simulink model "dspproject"  (R2025b)
settings: Solver=VariableStepAuto  StartTime=0.0  StopTime=10.0  RelTol=1e-3
undefined symbols (not defined in the file): dspblkCoreblockFVToolHelper, gcbh
libraries: audiofeatures x2, simulink x1, dspxfrm3 x1, dspsigops x1, dspvision x1
settings Model: Creator=BILMOOT  LastModifiedBy=BILMOOT

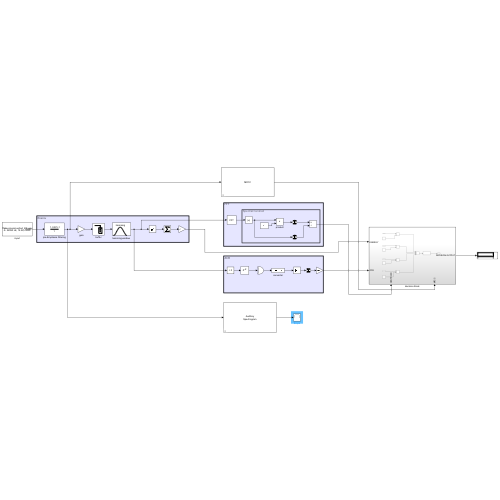
[thumbnail: Simulink's stored preview of the top-level diagram]
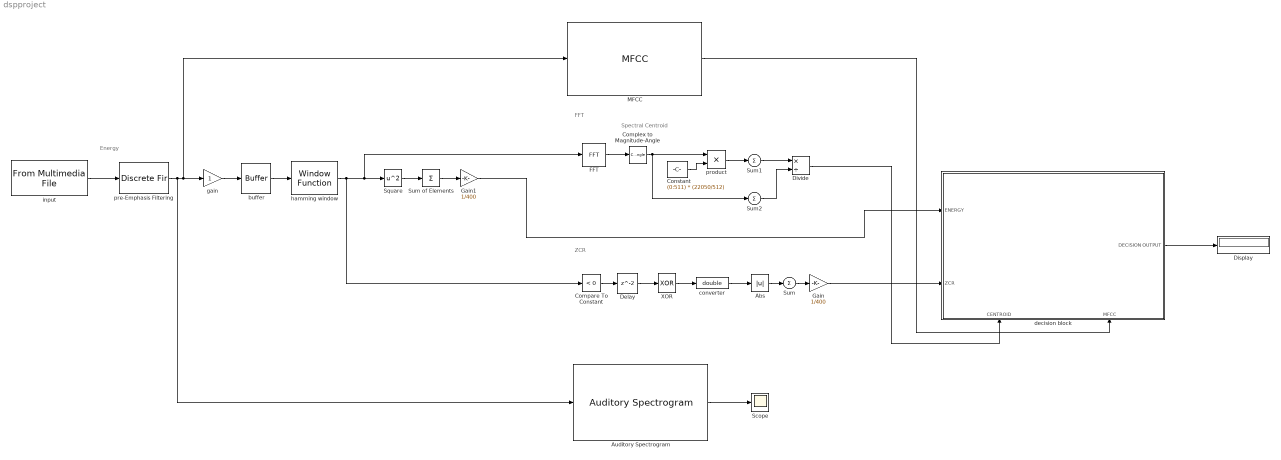
== system dspproject ==
  note: FFT
  note: Spectral Centroid
  note: Energy
  note: ZCR
  Abs : Abs  SaturateOnIntegerOverflow=off
  Auditory Spectrogram : audiofeatures/Auditory Spectrogram  FrequencyScale=mel  MelStyle=slaney  AutoNumBands=on  NumBands=32  AutoFrequencyRange=on  FrequencyRange=[0, 22050]  FilterBankDesignDomain=linear  FilterBankNormalization=bandwidth  OutputFrequencyVector=off  WindowParameter=hamming(400,'periodic')  WindowNormalization=on  OverlapLength=200  AutoFFTLength=on  FFTLength=1024  SpectrumType=magnitude  ApplyLog=off  NumHops=1  NumHopsOverlap=0  InheritSampleRate=on  SampleRate=44.1e3
  Compare To Constant : simulink/Logic and Bit Operations/Compare To Constant  relop=<  const=0  OutDataTypeStr=boolean
  Complex to Magnitude-Angle : ComplexToMagnitudeAngle  Output=Magnitude
  Constant : Constant  Value=(0:511) * (22050/512)
  Delay : Delay
  Display : Display
  Divide : Product  Inputs=*/
  FFT : dspxfrm3/FFT  FFTImplementation=Auto  CompMethod=Table lookup  TableOpt=NEW  TableOptActive=Speed  BitRevOrder=off  Normalize=on  InheritFFTLength=off  FFTLength=512  WrapInput=on  roundingMode=Round  overflowMode=on  firstCoeffDataTypeStr=Inherit: Same word length as input  firstCoeffLastDataTypeStr=Inherit: Same word length as input  outputMin=[]  outputMax=[]
  Gain : Gain  Gain=1/400
  Gain1 : Gain  Gain=1/400
  MFCC : audiofeatures/MFCC  WindowParameter=hamming(400,'periodic')  OverlapLength=200  NumCoeffs=13  Rectification=Logarithm  AppendDelta=on  AppendDeltaDelta=on  DeltaWindowLength=9  NumFeatureVectors=1  NumFeatureVectorOverlap=0  InheritSampleRate=off  SampleRate=22050  NumBands=26  AutoFrequencyRange=on  FrequencyRange=[0, 22050]  FilterBankDesignDomain=linear  FilterBankNormalization=bandwidth  MelStyle=slaney  WindowNormalization=on  SpectrumType=power  AutoFFTLength=on  FFTLength=1024
  Scope : Scope
      settings: ActiveDisplayYMinimum=-4.8863057234241722E-5  ActiveDisplayYMaximum=0.0004397675151081756
  Square : Math  Operator=square
  Sum : Sum  Inputs=+  CollapseMode=Specified dimension
  Sum of Elements : Sum  Inputs=+  CollapseMode=Specified dimension
  Sum1 : Sum  Inputs=+  CollapseMode=Specified dimension
  Sum2 : Sum  Inputs=+  CollapseMode=Specified dimension
  XOR : Logic  Operator=XOR  Inputs=1  IconShape=distinctive  AllPortsSameDT=off  OutDataTypeStr=boolean
  buffer : Buffer  N=400  V=240  OutputFrames=off
  converter : DataTypeConversion  OutDataTypeStr=double  SaturateOnIntegerOverflow=off  RndMeth=Floor
  decision block : Subsystem
      settings: PortSchema="{\"entries\":[{\"content\":{\"sides\":[{\"content\":{\"connectorIds\":[\"In1\",\"In2\"]},\"type\":\"ConnectorPlacement.EquallySpacedRectSide\",\"uuid\":\"88a2a444-5f90-4f1f-807a-bd703364281a\"},{\"content\":{\"connectorIds\":[\"Out1\"],\"side\":\"RIGHT\"},\"type\":\"ConnectorPlacement.EquallySpacedRectSide\",\"uuid\":\"4ec65e0f-1ccf-451e-b825-09269428c0b3\"},{\"content\":{\"side\":\"TOP\"},\"type\":\"ConnectorPlacement.EquallySpacedRectSide\",\"uuid\":\"c91968c7-69ce-4166-a477-17bcca02a99e\"},{\"content\":{\"connectorIds\":[\"In3\",\"In4\"],\"side\":\"BOTTOM\"},\"type\":\"ConnectorPlacement.EquallySpacedRectSide\",\"uuid\":\"9a55e096-9575-4f24-8ed3-8e9f0ae48f94\"}]},\"type\":\"ConnectorPlacement.EquallySpacedConnector\",\"uuid\":\"39e846e1-8f80-4fb5-8d1f-e6fff8928494\"}],\"packageUris\":[\"http://schema.mathworks.com/mf0/Connector/R2020b\"],\"version\":\"1.0\"}"
  gain : Gain
  "hamming window " : dspsigops/Window Function  winmode=Apply window to input  wintype=Hamming  sampmode=Continuous  samptime=1  N=64  Rs=50  beta=10  winsamp=Symmetric  UserWindow=hamming  OptParams=off  UserParams={'symmetric'}  dataType=double  isSigned=on  wordLen=16  udDataType=sfix(16)  fracBitsMode=Best precision  numFracBits=15  roundingMode=Nearest  overflowMode=on  numSidelobes=4  sidelobeLevel=-30
  input : dspvision/From Multimedia File  inputFilename=C:\Users\حاسبات الوادي\OneDrive\Documents\MATLAB\1fakevoiceconverted_22k.wav  readRange=[1 Inf]  loop=on  numPlays=inf  outputStreams=Audio only  videoDataType=single  audioDataType=double  inheritSampleTime=on  userDefinedSampleTime=1/30  noAudioOutput=off  isIntensityVideo=off  fourcc=RGB  colorVideoFormat=One multidimensional signal  outputEOF=off  dataOrg=Column-major  audioFrameSize=1024  computeAudioFrameSize=off  outSamplingMode=Sample based
      settings: LibrarySourceBlock=dspsrcs4/From Multimedia File
  pre-Emphasis Filtering : DiscreteFir  LoadFcn=dspblkCoreblockFVToolHelper(gcbh,'load');  Coefficients=[1 -0.97]  InputProcessing=Columns as channels (frame based)
      settings: CopyFcn=dspblkCoreblockFVToolHelper(gcbh,'copy');  DeleteFcn=dspblkCoreblockFVToolHelper(gcbh,'close');  ModelCloseFcn=dspblkCoreblockFVToolHelper(gcbh,'close');  PreSaveFcn=dspblkCoreblockFVToolHelper(gcbh,'presave');  PostSaveFcn=dspblkCoreblockFVToolHelper(gcbh,'postsave');  CloseFcn=dspblkCoreblockFVToolHelper(gcbh,'close');
  product : Product
  wires:
  gain/1 -> buffer/1
  Sum/1 -> Gain/1
  Compare To Constant/1 -> Delay/1
  Delay/1 -> XOR/1
  Abs/1 -> Sum/1
  input/1 -> pre-Emphasis Filtering/1
  "hamming window "/1 -> Compare To Constant/1, FFT/1, Square/1
  Square/1 -> Sum of Elements/1
  pre-Emphasis Filtering/1 -> Auditory Spectrogram/1, MFCC/1, gain/1
  Sum of Elements/1 -> Gain1/1
  FFT/1 -> Complex to Magnitude-Angle/1
  Complex to Magnitude-Angle/1 -> Sum2/1, product/1
  Constant/1 -> product/2
  product/1 -> Sum1/1
  Sum1/1 -> Divide/1
  Sum2/1 -> Divide/2
  Gain1/1 -> decision block/1(ENERGY)
  Gain/1 -> decision block/2(ZCR)
  Divide/1 -> decision block/3(CENTROID)
  MFCC/1 -> decision block/4(MFCC)
  XOR/1 -> converter/1
  converter/1 -> Abs/1
  decision block/1(DECISION OUTPUT) -> Display/1
  buffer/1 -> "hamming window "/1
  Auditory Spectrogram/1 -> Scope/1

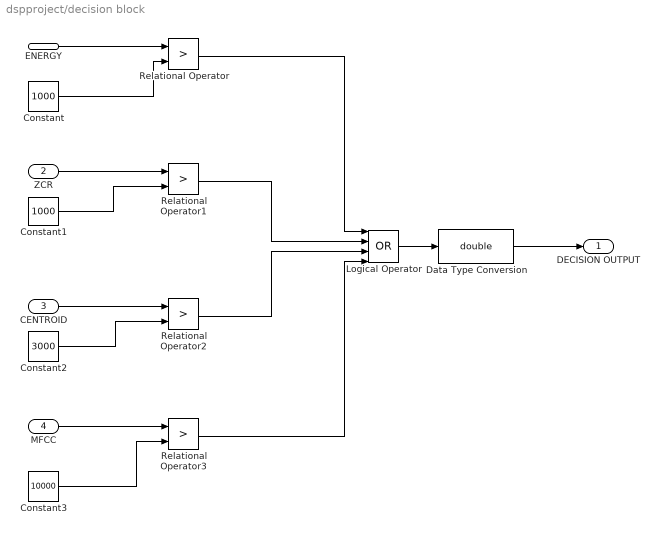
== system dspproject/decision block ==
  ENERGY : Inport
  ZCR : Inport  Port=2
  CENTROID : Inport  Port=3
  MFCC : Inport  Port=4
  Constant : Constant  Value=1000
  Constant1 : Constant  Value=1000
  Constant2 : Constant  Value=3000
  Constant3 : Constant  Value=10000
  Data Type Conversion : DataTypeConversion  OutDataTypeStr=double  SaturateOnIntegerOverflow=off  RndMeth=Floor
  Logical Operator : Logic  Operator=OR  Inputs=4  AllPortsSameDT=off  OutDataTypeStr=boolean
  Relational Operator{,1..3} (4 alike) : RelationalOperator  Operator=>  OutDataTypeStr=boolean  RndMeth=Simplest  InputSameDT=off
  DECISION OUTPUT : Outport  OutDataTypeStr=double
  wires:
  Constant/1 -> Relational Operator/2
  Constant1/1 -> Relational Operator1/2
  Constant2/1 -> Relational Operator2/2
  Data Type Conversion/1 -> DECISION OUTPUT/1
  Logical Operator/1 -> Data Type Conversion/1
  Constant3/1 -> Relational Operator3/2
  Relational Operator/1 -> Logical Operator/1
  CENTROID/1 -> Relational Operator2/1
  ENERGY/1 -> Relational Operator/1
  MFCC/1 -> Relational Operator3/1
  ZCR/1 -> Relational Operator1/1
  Relational Operator3/1 -> Logical Operator/4
  Relational Operator1/1 -> Logical Operator/2
  Relational Operator2/1 -> Logical Operator/3
